simulink model "Cruise_Control_System"  (R2018a)
settings: Solver=VariableStepAuto  StartTime=0.0  StopTime=100  RelTol=1e-3
libraries: simulink x1
settings Model: Creator=Acer  LastModifiedBy=Acer

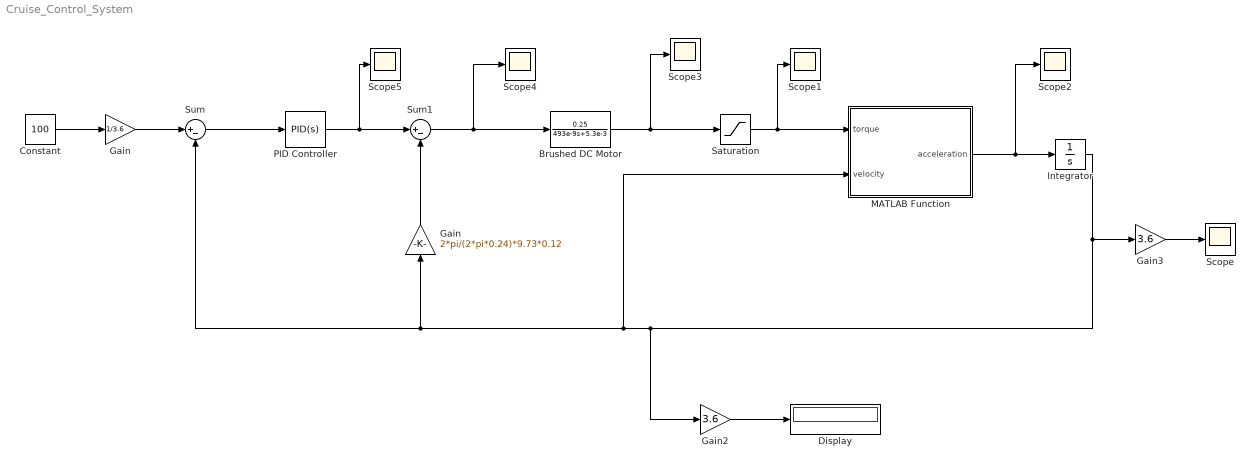
== system Cruise_Control_System ==
  "Brushed DC Motor " : TransferFcn  Numerator=[0.25]  Denominator=[493e-9 5.3e-3]
  Constant : Constant  Value=100
  Display : Display
  Gain : Gain  Gain=1/3.6
  "Gain " : Gain  Gain=2*pi/(2*pi*0.24)*9.73*0.12
  Gain2 : Gain  Gain=3.6
  Gain3 : Gain  Gain=3.6
  Integrator : Integrator
  MATLAB Function : MATLAB Function  TreatAsAtomicUnit=on
  "PID Controller " : simulink/Continuous/PID Controller  Controller=PID  TimeDomain=Continuous-time  SampleTime=-1  IntegratorMethod=Forward Euler  FilterMethod=Forward Euler  Form=Parallel  UseFilter=on  ControllerParametersSource=internal  P=1000  I=5  D=0  N=100  InitialConditionSource=internal  InitialConditionForIntegrator=0  InitialConditionForFilter=0  ExternalReset=none  LimitOutput=on  UpperSaturationLimit=346  LowerSaturationLimit=0  LinearizeAsGain=on  AntiWindupMode=none  Kb=1  TrackingMode=off  Kt=1  PParamMin=[]  PParamMax=[]  IParamMin=[]  IParamMax=[]  DParamMin=[]  DParamMax=[]  NParamMin=[]  NParamMax=[]  KbParamMin=[]  KbParamMax=[]  KtParamMin=[]  KtParamMax=[]  POutMin=[]  POutMax=[]  IOutMin=[]  IOutMax=[]  DOutMin=[]  DOutMax=[]  NOutMin=[]  NOutMax=[]  KbOutMin=[]  KbOutMax=[]  KtOutMin=[]  KtOutMax=[]  IntegratorOutMin=[]  IntegratorOutMax=[]  FilterOutMin=[]  FilterOutMax=[]  SumOutMin=[]  SumOutMax=[]  SumI1OutMin=[]  SumI1OutMax=[]  SumI2OutMin=[]  SumI2OutMax=[]  SumI3OutMin=[]  SumI3OutMax=[]  SumDOutMin=[]  SumDOutMax=[]  SaturationOutMin=[]  SaturationOutMax=[]  IntegratorContinuousStateAttributes=''  IntegratorStateMustResolveToSignalObject=off  IntegratorRTWStateStorageClass=Auto  FilterContinuousStateAttributes=''  FilterStateMustResolveToSignalObject=off  FilterRTWStateStorageClass=Auto  DifferentiatorICPrevScaledInput=0  DifferentiatorOutMin=[]  DifferentiatorOutMax=[]  FilterDiffOutCoefMin=[]  FilterDiffOutCoefMax=[]  SumDenOutMin=[]  SumDenOutMax=[]  SumNumOutMin=[]  SumNumOutMax=[]  ReciprocalOutMin=[]  ReciprocalOutMax=[]  DivideOutMin=[]  DivideOutMax=[]  TunerSelectOption=Transfer Function Based (PID Tuner App)
  Saturation : Saturate  UpperLimit=601  LowerLimit=0
  Scope{,1..5} (6 alike) : Scope
  Sum : Sum  Inputs=|+-
  Sum1 : Sum  Inputs=|+-
  wires:
  Constant/1 -> Gain/1
  Gain/1 -> Sum/1
  Sum/1 -> "PID Controller "/1
  "PID Controller "/1 -> Scope5/1, Sum1/1
  "Gain "/1 -> Sum1/2
  Sum1/1 -> Scope4/1, "Brushed DC Motor "/1
  Saturation/1 -> Scope1/1, MATLAB Function/1(torque)
  MATLAB Function/1(acceleration) -> Scope2/1, Integrator/1
  Gain2/1 -> Display/1
  Gain3/1 -> Scope/1
  Integrator/1 -> Gain3/1, Gain2/1, Sum/2, "Gain "/1, MATLAB Function/2(velocity)
  "Brushed DC Motor "/1 -> Scope3/1, Saturation/1

== matlab function Cruise_Control_System/MATLAB Function ==
  data: torque input; acceleration output; velocity input
function acceleration = fcn(torque,velocity)
acceleration = (40.5*torque*0.7-413-0.3381*velocity^2)/2108;
